simulink model "test_ZieglerNichols"  (R2024a)
settings: Solver=VariableStepAuto  StartTime=0.0  StopTime=300  RelTol=1e-3
settings Model: Creator=neerz  LastModifiedBy=neerz

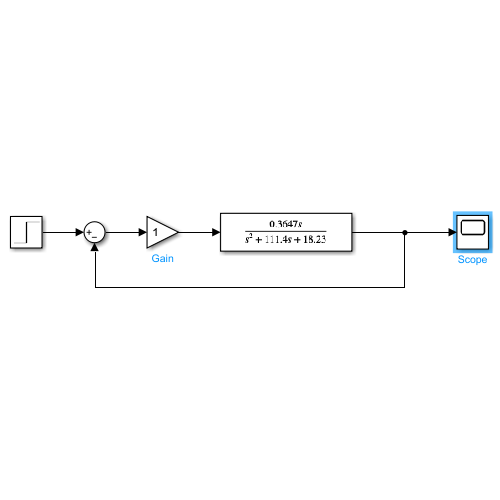
[thumbnail: Simulink's stored preview of the top-level diagram]
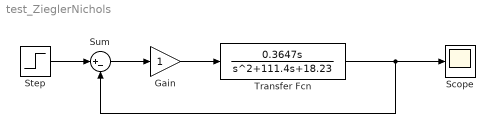
== system test_ZieglerNichols ==
  Gain : Gain
  Scope : Scope
  Step : Step  SampleTime=0
  Sum : Sum  Inputs=|+-
  Transfer Fcn : TransferFcn  Numerator=[0.3647 0]  Denominator=[1 111.4 18.23]
  wires:
  Gain/1 -> Transfer Fcn/1
  Sum/1 -> Gain/1
  Transfer Fcn/1 -> Sum/2, Scope/1
  Step/1 -> Sum/1
